simulink model "BeamLoading"  (R2022b)
settings: Solver=VariableStepAuto  StartTime=0.0  StopTime=10.0  RelTol=1e-3
settings Model: Creator=mliu  LastModifiedBy=mliu

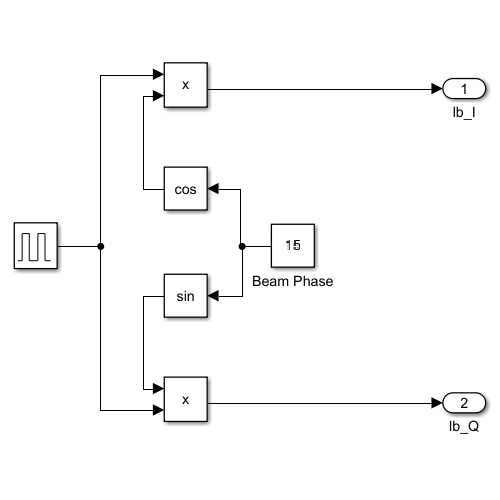
[thumbnail: Simulink's stored preview of the top-level diagram]
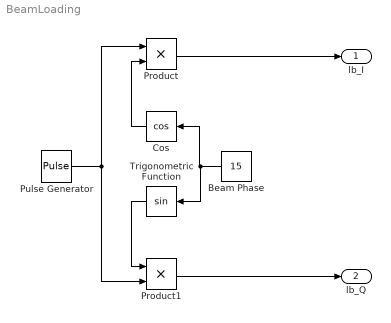
== system BeamLoading ==
  Beam Phase : Constant  Value=15
  Cos : Trigonometry  Operator=cos
  Product : Product
  Product1 : Product
  Pulse Generator : DiscretePulseGenerator  PulseType=Time based  Period=0.04  PulseWidth=5
  Trigonometric Function : Trigonometry
  lb_I : Outport
  lb_Q : Outport  Port=2
  wires:
  Pulse Generator/1 -> Product/1, Product1/2
  Cos/1 -> Product/2
  Trigonometric Function/1 -> Product1/1
  Beam Phase/1 -> Trigonometric Function/1, Cos/1
  Product/1 -> lb_I/1
  Product1/1 -> lb_Q/1
